simulink model "InterfaceGUI"  (R2024a)
settings: Solver=VariableStepAuto  StartTime=0.0  StopTime=10.0  RelTol=1e-3
values from neighbouring files (symbols this model uses):
  M_vector = [M_1; 0; 0]    [PARAMS_GUI.m]
  material_properties = [E_x.value, E_y.value, E_s.value, nu_x.value, nu_y.value, m.value, X_t.value, X_c.value, Y_t.value, Y_c.value, S_c.value, h_o.value, rho.value]    [PARAMS_GUI.m]
  N_vector = [N_1; 0; 0]    [PARAMS_GUI.m]
  schedule_base = [0, 0, 20, -20, 0, 90]    [PARAMS_GUI.m]
  symmetrical = true    [DESIGN_1_Interface.m]    (also in DESIGN_2_Interface_10.m; DESIGN_2_Interface_Preloop.m; PARAMS_GUI.m)
  z_c = 0.005    [DESIGN3_Test1.m]    (also in DESIGN3_Test2.m; DESIGN_1_Interface.m; DESIGN_2_Interface_10.m = 0; DESIGN_2_Interface_10_20.m = 0)
settings Model: Creator=phil  LastModifiedBy=phil

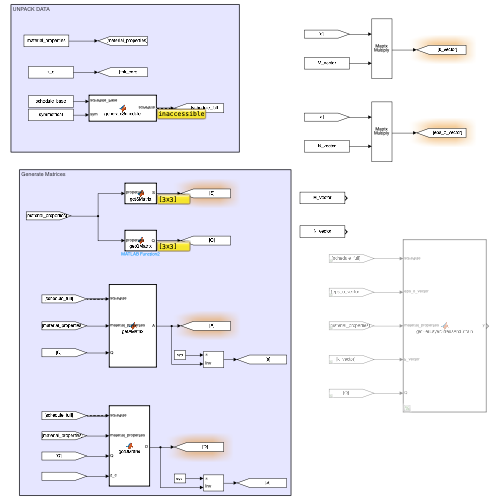
[thumbnail: Simulink's stored preview of the top-level diagram]
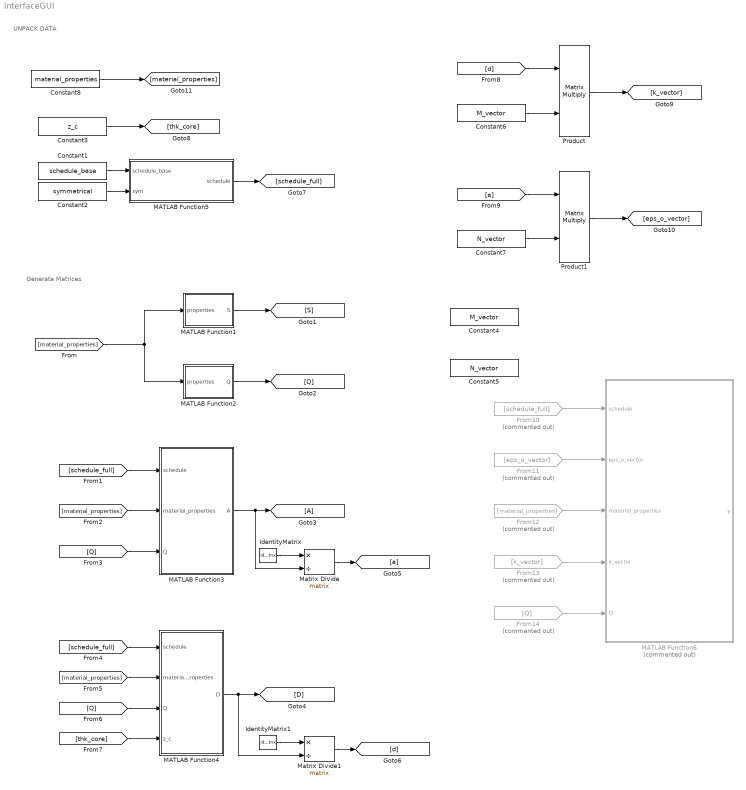
== system InterfaceGUI ==
  note: Generate Matrices
  note: UNPACK DATA
  Constant1 : Constant  Value=schedule_base
  Constant2 : Constant  Value=symmetrical
  Constant3 : Constant  Value=z_c
  Constant4 : Constant  Value=M_vector
  Constant5 : Constant  Value=N_vector
  Constant6 : Constant  Value=M_vector
  Constant7 : Constant  Value=N_vector
  Constant8 : Constant  Value=material_properties
  From10 : From  Commented=on  GotoTag=schedule_full
  From11 : From  Commented=on  GotoTag=eps_o_vector
  From12 : From  Commented=on  GotoTag=material_properties
  From13 : From  Commented=on  GotoTag=k_vector
  From14 : From  Commented=on  GotoTag=Q
  Goto3 : Goto
  IdentityMatrix : IdentityMatrix  OutputDimensions=3
  IdentityMatrix1 : IdentityMatrix  OutputDimensions=3
  MATLAB Function1 : MATLAB Function  TreatAsAtomicUnit=on
  MATLAB Function2 : MATLAB Function  TreatAsAtomicUnit=on
  MATLAB Function3 : MATLAB Function  TreatAsAtomicUnit=on
  MATLAB Function4 : MATLAB Function  TreatAsAtomicUnit=on
  MATLAB Function5 : MATLAB Function  TreatAsAtomicUnit=on
  MATLAB Function6 : MATLAB Function  Commented=on  TreatAsAtomicUnit=on
  Matrix Divide : Product  Inputs=*/  Multiplication=Matrix(*)
  Matrix Divide1 : Product  Inputs=*/  Multiplication=Matrix(*)
  Product : Product  Multiplication=Matrix(*)
  Product1 : Product  Multiplication=Matrix(*)
  wires:
  MATLAB Function3/1(A) -> Matrix Divide/2, Goto3/1
  MATLAB Function4/1(D) -> Matrix Divide1/2, [D]
  [material_properties] -> MATLAB Function1/1(properties), MATLAB Function2/1(properties)
  MATLAB Function1/1(S) -> [S]
  MATLAB Function2/1(Q) -> [Q]
  Constant1/1 -> MATLAB Function5/1(schedule_base)
  Constant2/1 -> MATLAB Function5/2(sym)
  MATLAB Function5/1(schedule) -> [schedule_full]
  [schedule_full] -> MATLAB Function3/1(schedule)
  [Q] -> MATLAB Function3/3(Q)
  [material_properties] -> MATLAB Function3/2(material_properties)
  [schedule_full] -> MATLAB Function4/1(schedule)
  [material_properties] -> MATLAB Function4/2(material_properties)
  [Q] -> MATLAB Function4/3(Q)
  [thk_core] -> MATLAB Function4/4(z_c)
  Constant3/1 -> [thk_core]
  Product/1 -> [k_vector]
  Product1/1 -> [eps_o_vector]
  [d] -> Product/1
  [a] -> Product1/1
  Constant6/1 -> Product/2
  Constant7/1 -> Product1/2
  From10/1 -> MATLAB Function6/1(schedule)
  From11/1 -> MATLAB Function6/2(eps_o_vector)
  From12/1 -> MATLAB Function6/3(material_properties)
  From13/1 -> MATLAB Function6/4(k_vector)
  From14/1 -> MATLAB Function6/5(Q)
  Constant8/1 -> [material_properties]
  Matrix Divide/1 -> [a]
  IdentityMatrix/1 -> Matrix Divide/1
  IdentityMatrix1/1 -> Matrix Divide1/1
  Matrix Divide1/1 -> [d]

== matlab function InterfaceGUI/MATLAB Function1 ==
  data: properties input; S output
function S = getSMatrix(properties)

E_x = properties(1);
E_y = properties(2);
E_s = properties(3);
nu_x = properties(4);
nu_y = properties(5);

S_xx = 1 / E_x;
S_xy = -nu_y / E_y;
S_yx = -nu_x / E_x;
S_yy = 1 / E_y;
S_ss = 1 / E_s;

S = [S_xx, S_xy, 0; 
     S_yx, S_yy, 0; 
     0,    0,    S_ss];

== matlab function InterfaceGUI/MATLAB Function2 ==
  data: properties input; Q output
function Q = getQMatrix(properties)

E_x = properties(1);
E_y = properties(2);
E_s = properties(3);
nu_x = properties(4);
nu_y = properties(5);
m = properties(6);

% Compute stiffness coefficients
Q_xx = m * E_x;
Q_yy = m * E_y;
Q_yx = m * nu_x * E_y;
Q_xy = m * nu_y * E_x;
Q_ss = E_s;

% Form the stiffness matrix
Q = [Q_xx, Q_xy, 0; 
     Q_yx, Q_yy, 0; 
     0,    0,    Q_ss];

== matlab function InterfaceGUI/MATLAB Function3 ==
  data: schedule input; A output; material_properties input; Q input
function A = getAMatrix(schedule, material_properties, Q)

h = material_properties(12);

A = calculateAMatrix(schedule, h, Q);

== matlab function InterfaceGUI/MATLAB Function4 ==
  data: schedule input; D output; material_properties input; Q input; z_c input
function D = getDMatrix(schedule, material_properties, Q, z_c)

h = material_properties(12);

D = calculateDMatrix(schedule, h, Q, z_c);

== matlab function InterfaceGUI/MATLAB Function5 ==
  data: schedule_base input; schedule output; sym input
function schedule = generateSchedule(schedule_base, sym)

if sym
    % Create symmetric schedule
    schedule = [schedule_base, fliplr(schedule_base)];
else
    % Return the base schedule
    schedule = schedule_base;
end

== matlab function InterfaceGUI/MATLAB Function6 ==
  data: schedule input; y output; eps_o_vector input; material_properties input; k_vector input; Q input
function y = getPerLayerStressAndStrain(schedule, eps_o_vector, material_properties, k_vector, Q)

y = u;
